simulink model "ADAS_Simulink_Model_HIL"  (R2026a)
settings: Solver=FixedStepDiscrete  FixedStep=0.1
undefined symbols (not defined in the file or in its folder): canChannel
libraries: canlib x4, simulink x3, canmsglib x2
settings Model: Creator=mushu  LastModifiedBy=mushu

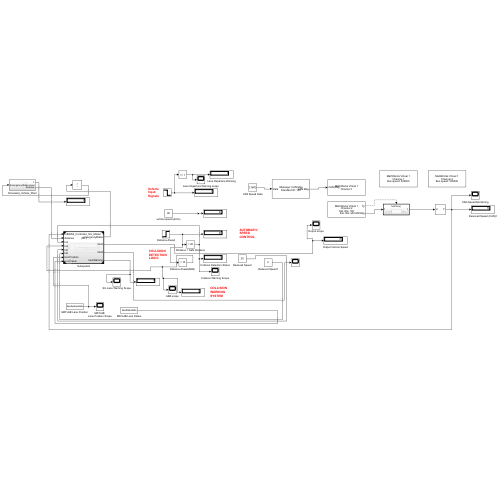
[thumbnail: Simulink's stored preview of the top-level diagram]
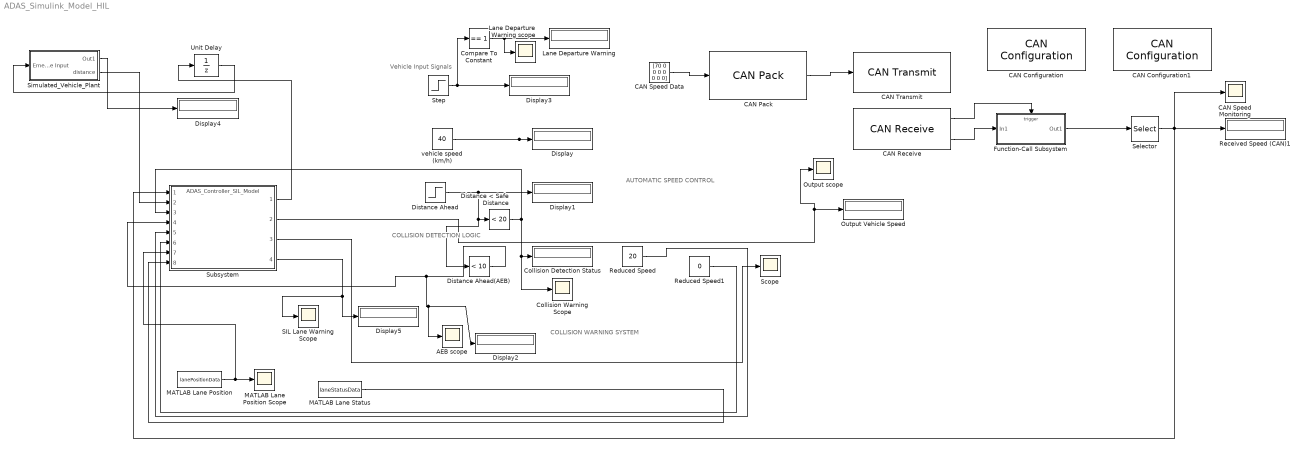
== system ADAS_Simulink_Model_HIL ==
  note: COLLISION WARNING SYSTEM
  note: AUTOMATIC SPEED CONTROL
  note: COLLISION DETECTION LOGIC
  note: Vehicle Input Signals
  AEB scope : Scope
      settings: ActiveDisplayYMinimum=-0.12499999999999997  ActiveDisplayYMaximum=1.125  DataLoggingVariableName=ScopeData4
  CAN Configuration : canlib/CAN Configuration  BlockHandle=154.0001  Device=MathWorks Virtual 1 (Channel 1)  DeviceMenu=MathWorks Virtual 1 (Channel 1)  ObjConstructor=canChannel('MathWorks', 'Virtual 1', 1)  BusSpeed=500000  EnableBitParameters=off  AckMode=Normal
  CAN Configuration1 : canlib/CAN Configuration  BlockHandle=155.0001  Device=MathWorks Virtual 1 (Channel 2)  DeviceMenu=MathWorks Virtual 1 (Channel 2)  ObjConstructor=canChannel('MathWorks', 'Virtual 1', 2)  BusSpeed=500000  EnableBitParameters=off  AckMode=Normal
  CAN Pack : canmsglib/CAN Pack  MsgList=(none)  MsgName=CAN Msg  MsgIDType=Standard (11-bit identifier)  MsgIdentifier=100  CANIDInput=off  MsgLength=8  Remote=off  ApplyMinMax=off  BusOutput=off  SignalInfo={}
      settings: LibrarySourceBlock=canlib/CAN Pack  DataFormat=raw data
  CAN Receive : canlib/CAN Receive  BlockHandle=159.0001  Device=MathWorks Virtual 1 (Channel 2)  DeviceMenu=MathWorks Virtual 1 (Channel 2)  ObjConstructor=canChannel('MathWorks', 'Virtual 1', 2)  EnableStandardIDsFilter=off  StdIDsCombo=Allow only  StandardIDs=100  EnableExtendedIDsFilter=off  ExtIDsCombo=Allow all  ExtendedIDs=0  SampleTime=0.1  MsgsPerTimestep=all  InternalFilterUpdateStatus=on  BusOutput=off
  CAN Speed Data : Constant  Value=[70 0 0 0 0 0 0 0]  VectorParams1D=off  OutDataTypeStr=uint8  SampleTime=0.1
  CAN Speed Monitoring : Scope
      settings: ActiveDisplayYMinimum=-1  ActiveDisplayYMaximum=1  DataLoggingVariableName=ScopeData5
  CAN Transmit : canlib/CAN Transmit  BlockHandle=294.0001  Device=MathWorks Virtual 1 (Channel 1)  DeviceMenu=MathWorks Virtual 1 (Channel 1)  ObjConstructor=canChannel('MathWorks', 'Virtual 1', 1)  EnableEventTransmit=off  EnablePeriodicTransmit=off  MessagePeriod=0.1
  Collision Detection Status : Display
  Collision Warning Scope : Scope
      settings: ActiveDisplayYMinimum=-1  ActiveDisplayYMaximum=1
  Compare To Constant : simulink/Logic and Bit Operations/Compare To Constant  relop===  const=1  OutDataTypeStr=boolean
  Display{,1..5} (6 alike) : Display
  Distance < Safe Distance : simulink/Logic and Bit Operations/Compare To Constant  relop=<  const=20  OutDataTypeStr=boolean
  Distance Ahead : Step  Time=3  InitialValue=25  FinalValue=25  SampleTime=0
  "Distance Ahead(AEB) " : simulink/Logic and Bit Operations/Compare To Constant  relop=<  const=10  OutDataTypeStr=boolean
  Function-Call Subsystem : Subsystem  TreatAsAtomicUnit=on
  Lane Departure Warning : Display
  Lane Departure Warning scope : Scope
      settings: ActiveDisplayYMinimum=0.92006938414883432  ActiveDisplayYMaximum=1.1450709232422684  DataLoggingVariableName=ScopeData3
  MATLAB Lane Position Scope : Scope
      settings: ActiveDisplayYMinimum=-1.25  ActiveDisplayYMaximum=1.25  DataLoggingVariableName=ScopeData7
  MATLAB Lane Position : FromWorkspace  VariableName=lanePositionData  SampleTime=0.1  Interpolate=off  OutputAfterFinalValue=Holding final value
  MATLAB Lane Status : FromWorkspace  VariableName=laneStatusData  Interpolate=off  OutputAfterFinalValue=Holding final value
  Output Vehicle Speed : Display
  Output scope : Scope
      settings: ActiveDisplayYMinimum=-1  ActiveDisplayYMaximum=1  DataLoggingVariableName=ScopeData2
  Received Speed (CAN)1 : Display
  Reduced Speed : Constant  Value=20
  Reduced Speed1 : Constant  Value=0
  SIL Lane Warning Scope : Scope
      settings: ActiveDisplayYMinimum=-2.1720070431317877  ActiveDisplayYMaximum=3.3999181376715004  DataLoggingVariableName=ScopeData6
  Scope : Scope
      settings: ActiveDisplayYMinimum=17.5  ActiveDisplayYMaximum=42.5
  Selector : Selector  InputPortWidth=8  IndexOptions=Index vector (dialog)  Indices=1  OutputSizes=1
  Simulated_Vehicle_Plant : Subsystem
  Step : Step  Time=5  InitialValue=1  FinalValue=0  SampleTime=0
  Subsystem : ModelReference  ModelNameDialog=ADAS_Controller_SIL_Model  SimulationMode=Software-in-the-loop (SIL)  ModelReferenceVersion=1.115
  Unit Delay : UnitDelay  SampleTime=0.1
  vehicle speed (km/h) : Constant  Value=40
  wires:
  vehicle speed (km/h)/1 -> Display/1
  Distance Ahead/1 -> "Distance Ahead(AEB) "/1, Distance < Safe Distance/1, Display1/1
  Distance < Safe Distance/1 -> Subsystem/3, Collision Warning Scope/1, Collision Detection Status/1
  "Distance Ahead(AEB) "/1 -> Subsystem/4, AEB scope/1, Display2/1
  Step/1 -> Compare To Constant/1, Display3/1
  Compare To Constant/1 -> Lane Departure Warning scope/1, Lane Departure Warning/1
  CAN Pack/1 -> CAN Transmit/1
  CAN Speed Data/1 -> CAN Pack/1
  MATLAB Lane Position/1 -> Subsystem/7, MATLAB Lane Position Scope/1
  Function-Call Subsystem/1(Out1) -> Selector/1
  CAN Receive/2 -> Function-Call Subsystem/1(In1)
  CAN Receive/1 -> Function-Call Subsystem/Trigger
  Subsystem/4 -> SIL Lane Warning Scope/1, Display5/1
  Subsystem/2 -> Output scope/1, Output Vehicle Speed/1
  Reduced Speed/1 -> Subsystem/5
  Reduced Speed1/1 -> Subsystem/6
  MATLAB Lane Status/1 -> Subsystem/8
  Subsystem/3 -> Scope/1
  Simulated_Vehicle_Plant/2(distance) -> Subsystem/2
  Subsystem/1 -> Unit Delay/1
  Unit Delay/1 -> Simulated_Vehicle_Plant/1(Emergency Brake Input)
  Selector/1 -> CAN Speed Monitoring/1, Subsystem/1, Received Speed (CAN)1/1
  Simulated_Vehicle_Plant/1(Out1) -> Display4/1

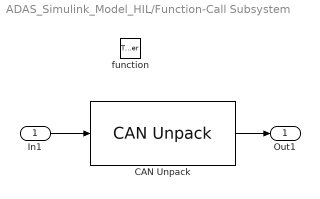
== system ADAS_Simulink_Model_HIL/Function-Call Subsystem ==
  In1 : Inport
  function : TriggerPort  TriggerType=function-call  VariantControl=(inherit)
  CAN Unpack : canmsglib/CAN Unpack  MsgList=(none)  MsgName=CAN Msg  MsgIDType=Standard (11-bit identifier)  MsgIdentifier=100  MsgLength=8  SignalInfo={}  IDPort=off  TimestampPort=off  ErrorPort=off  RemotePort=off  LengthPort=off  StatusPort=off  ApplyMinMax=off
      settings: LibrarySourceBlock=canlib/CAN Unpack  DataFormat=raw data
  Out1 : Outport
  wires:
  CAN Unpack/1 -> Out1/1
  In1/1 -> CAN Unpack/1

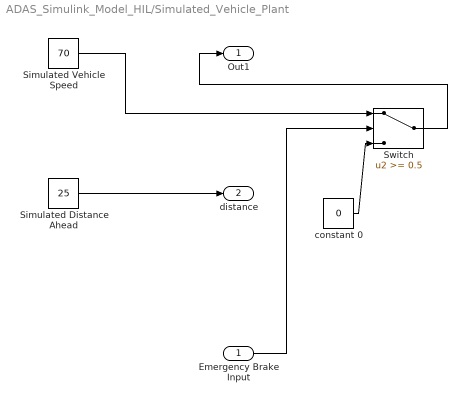
== system ADAS_Simulink_Model_HIL/Simulated_Vehicle_Plant ==
  Emergency Brake Input : Inport  SampleTime=0.1
  Simulated Distance Ahead : Constant  Value=25  VectorParams1D=off  SampleTime=0.1
  Simulated Vehicle Speed : Constant  Value=70  VectorParams1D=off  SampleTime=0.1
  Switch : Switch  Threshold=0.5  SaturateOnIntegerOverflow=off  InputSameDT=off
  constant 0 : Constant  Value=0  VectorParams1D=off  SampleTime=0.1
  Out1 : Outport
  distance : Outport  Port=2
  wires:
  Simulated Distance Ahead/1 -> distance/1
  Simulated Vehicle Speed/1 -> Switch/1
  constant 0/1 -> Switch/3
  Emergency Brake Input/1 -> Switch/2
  Switch/1 -> Out1/1
